simulink model "Traffic_moore"  (R2020b)
settings: Solver=FixedStepDiscrete  StartTime=0.0  StopTime=150  FixedStep=0.1  RelTol=1e-3
undefined symbols (not defined in the file): DiscIntNeverNeededParam
libraries: simulink x1
settings Model: EnablePacing=on  PacingRate=4  Creator=shivanshu shukla  LastModifiedBy=shivanshu shukla

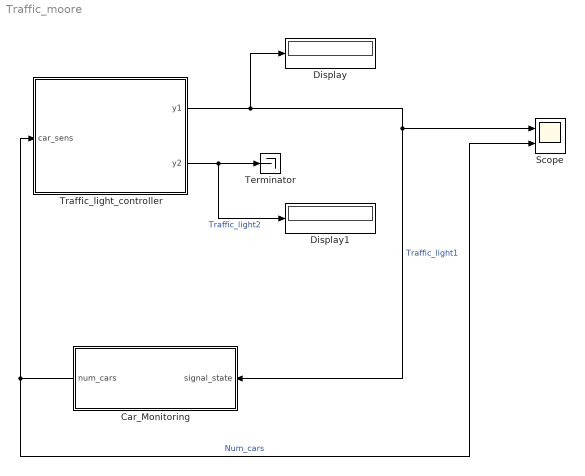
== system Traffic_moore ==
  Car_Monitoring : Subsystem
  Display : Display
  Display1 : Display
  Scope : Scope  NumInputPorts=2
  Terminator : Terminator
  Traffic_light_controller : Stateflow chart  TreatAsAtomicUnit=on
  wires:
  Traffic_light_controller/1(y1) -> Display/1, Scope/1, Car_Monitoring/1(signal_state)  "Traffic_light1"
  Traffic_light_controller/2(y2) -> Display1/1, Terminator/1  "Traffic_light2"
  Car_Monitoring/1(num_cars) -> Traffic_light_controller/1(car_sens), Scope/2  "Num_cars"

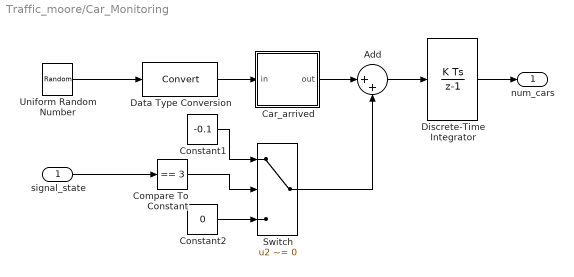
== system Traffic_moore/Car_Monitoring ==
  signal_state : Inport
  Add : Sum  Inputs=|++
  Car_arrived : Stateflow chart  TreatAsAtomicUnit=on
  Compare To Constant : simulink/Logic and Bit Operations/Compare To Constant  relop===  const=3  OutDataTypeStr=boolean  ZeroCross=off
  Constant1 : Constant  Value=-0.1
  Constant2 : Constant  Value=0
  Data Type Conversion : DataTypeConversion
  Discrete-Time Integrator : DiscreteIntegrator  SampleTime=-1  LimitOutput=on  LowerSaturationLimit=0  ICPrevOutput=DiscIntNeverNeededParam  ICPrevScaledInput=DiscIntNeverNeededParam
  Switch : Switch  Criteria=u2 ~= 0
  Uniform Random Number : UniformRandomNumber  Minimum=0  Maximum=100  Seed=177836  SampleTime=0
  num_cars : Outport  VectorParamsAs1DForOutWhenUnconnected=off
  wires:
  Discrete-Time Integrator/1 -> num_cars/1
  Data Type Conversion/1 -> Car_arrived/1(in)
  Car_arrived/1(out) -> Add/1
  Constant1/1 -> Switch/1
  signal_state/1 -> Compare To Constant/1
  Uniform Random Number/1 -> Data Type Conversion/1
  Add/1 -> Discrete-Time Integrator/1
  Constant2/1 -> Switch/3
  Compare To Constant/1 -> Switch/2
  Switch/1 -> Add/2

== stateflow chart Traffic_moore/Traffic_light_controller ==
  settings: stateMachineType=MOORE_MACHINE  initializeOutput=1
  state Stop
    y1=RED;
    y2=GREEN;
  state StopForTraffic
    y1=RED;
    y2=GREEN;
  state StepToGo
    y1=RED;
    y2=YELLOW;
  state GoToStop
    y1=GREEN;
    y2=YELLOW;
  state Go
    y1=GREEN;
    y2=RED;
  (default) -> Stop
  Stop -> StopForTraffic : after(30,tick)
  StopForTraffic -> StepToGo : [car_sens]
  GoToStop -> Stop : after(4,tick)
  StepToGo -> Go : after(4,tick)
  Go -> GoToStop : after(15,tick)
  data: car_sens input double; y1 output double; y2 output double; GREEN constant double =3; RED constant uint8 =1; YELLOW constant double =2

== stateflow chart Traffic_moore/Car_Monitoring/Car_arrived ==
  (default) -> (junction 2) : {out = in > 98;}
  data: in input int8; out output double
